simulink model "HvCoorn"  (R2022b)
settings: configuration reference "Icar05FusaMdlCfg" (kept outside this file)
undefined symbols (not defined in the file): BMSActSt_ACChrg, BMSActSt_DCChrg, BMSActSt_disconnect, BMSActSt_offline, BMSActSt_online, BMSActSt_undefined, BMSMainNegRlySt_Clsd_SC, BMSMainNegRlySt_Open_SC, BMSMainNegRlySt_StuckInClsd_SC, BMSMainNegRlySt_StuckInOpen_SC, BMSMainPosRlySt_Clsd_SC, BMSMainPosRlySt_Open_SC, BMSMainPosRlySt_StuckInClsd_SC, BMSPrecRlySt_StuckInOpen_SC, BMSReqSt_ACChrg, BMSReqSt_DCChrg, BMSReqSt_emergencyOffline, BMSReqSt_offline, BMSReqSt_online, Chrg_stCycleBookMod_SC, Chrg_stSingleBookMod_SC, CmpgMod_stInactv_SC, DCDCActSt_buck, DCDCActSt_connected, DCDCActSt_disconnected, DCDCReqSt_buck, DCDCReqSt_standby, EngStrtStop_RefuModDft_SC, EPBActSt_Appld_SC, GearLvr_stDrvGearD_SC, GearLvr_stDrvGearN_SC, GearLvr_stDrvGearP_SC, GearLvr_stDrvGearR_SC, hpp_bACChargeLinkIni_C, hpp_bACChargeLinkOKIni_C, hpp_bAcChgEnaIni_C, hpp_bAcChgPauseIni_C, hpp_bAcLinkTempErrIni_C, hpp_bBattWarmReqIni_C, hpp_bHvilHwErrIni_C, hpp_bHvilStOkIni_C, hpp_bHvRelayClsActIni_C, hpp_bHvRelayOpnActIni_C, hpp_bHvRelayStuckIni_C, hpp_bParked4ChDchgIni_C, hpp_bRemLvBatMntnReqIni_C, hpp_bStartUpReqIni_C, hpp_stHvilCanIni_C, hpp_stWarmTimeCfgRespIni_C, HvCoorn_bAuthEnaSwt_C, HvCoorn_bAuthFailSpdLimOvrd_C, HvCoorn_bAuthFailSpdLimOvrdVal_C, HvCoorn_bAuthStrt_C, HvCoorn_bBMSUnexpdDcnctFailEna_C, HvCoorn_bBuck2RdyBypDCDCEna_C, HvCoorn_bDCChrgFctCfg_C, HvCoorn_bDcChrgWkupEnaChrgLink_C, HvCoorn_bDCDcnct4ACEna_C, HvCoorn_bDCNotBuck2ShtdwnEna_C, HvCoorn_bDrvrLevNotRdyEna_C ... (+295)
libraries: ITKLib x213, simulink x61
(part 2 of 12)

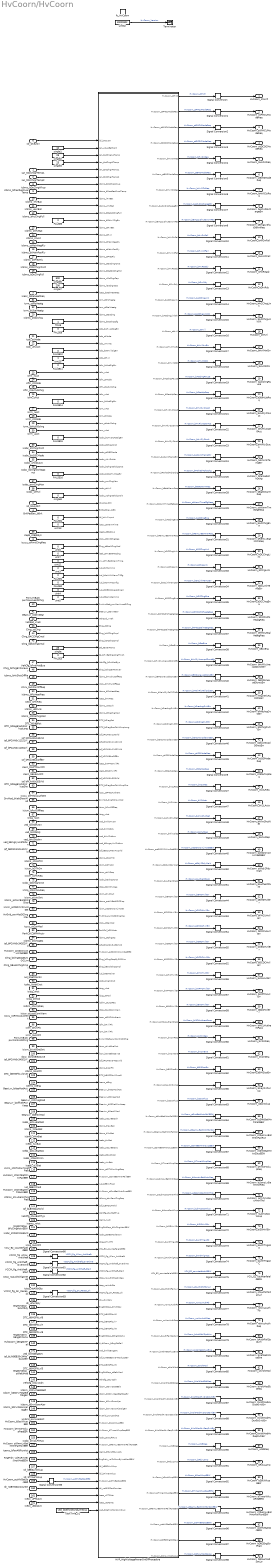
== system HvCoorn/HvCoorn ==
  ian_tDcChrgrTemp1 : Inport  OutDataTypeStr=single  Unit=deg
  ian_tDcChrgrTemp2 : Inport  Port=2  OutDataTypeStr=single  Unit=deg
  iczcu_stRmtChrgReq : Inport  Port=3  Unit=flg
  BrkPedDev_bBrk : Inport  Port=4  OutDataTypeStr=boolean  Unit=flg
  idi_bKeyStrt : Inport  Port=5  OutDataTypeStr=boolean  Unit=flg
  idi_bKeyOn : Inport  Port=6  OutDataTypeStr=boolean  Unit=flg
  icecc_bStalHeatReq : Inport  Port=7  OutDataTypeStr=boolean
  icbms_bDcChrgWkup : Inport  Port=8  OutDataTypeStr=boolean  Unit=flg
  icbms_bPrecResOverTemp : Inport  Port=9  OutDataTypeStr=boolean  Unit=flg
  icbms_iHVBat : Inport  Port=10  OutDataTypeStr=single  Unit=A
  icbms_uHVBat : Inport  Port=11  OutDataTypeStr=single  Unit=V
  icbms_bAcChrgFull : Inport  Port=12  OutDataTypeStr=boolean  Unit=flg
  icbms_stHvBat : Inport  Port=13  OutDataTypeStr=uint8
  icbms_stHvil : Inport  Port=14  OutDataTypeStr=uint8
  icbms_stMainNegRly : Inport  Port=15  OutDataTypeStr=uint8
  icbms_stMainPosRly : Inport  Port=16  OutDataTypeStr=uint8
  icbms_stPrecRly : Inport  Port=17  OutDataTypeStr=uint8
  icbms_stDcChrgrCnct : Inport  Port=18  OutDataTypeStr=uint8
  icbms_bDcChrgFull : Inport  Port=19  OutDataTypeStr=boolean  Unit=flg
  icbms_stDcChrg : Inport  Port=20
  icdc_stMode : Inport  Port=21  OutDataTypeStr=uint8
  icdc_uHvAct : Inport  Port=22  OutDataTypeStr=single  Unit=V
  icfm_nAct : Inport  Port=23  OutDataTypeStr=single  Unit=rpm
  icfm_stMode : Inport  Port=24  OutDataTypeStr=uint8
  icfm_stActvDchrg : Inport  Port=25  OutDataTypeStr=uint8
  icfm_uAct : Inport  Port=26  OutDataTypeStr=single  Unit=V
  icrm_nAct : Inport  Port=27  OutDataTypeStr=single  Unit=rpm
  icrm_stMode : Inport  Port=28  OutDataTypeStr=uint8
  icrm_stActvDchrg : Inport  Port=29  OutDataTypeStr=uint8
  icrm_uAct : Inport  Port=30  OutDataTypeStr=single  Unit=V
  icrm_stPlsHeatg : Inport  Port=31  OutDataTypeStr=uint8
  icrm_stStalHeatg : Inport  Port=32  OutDataTypeStr=uint8
  icobc_stChrgrCnct : Inport  Port=33  OutDataTypeStr=uint8
  icobc_stOBCMode : Inport  Port=34  OutDataTypeStr=uint8
  icobc_uHvDcAct : Inport  Port=35  OutDataTypeStr=single  Unit=V
  icobc_bChrgrCtrlSigCnct : Inport  Port=36
  icobc_pwrChrgMax : Inport  Port=37  OutDataTypeStr=single  Unit=W
  icobc_stHvil : Inport  Port=38  OutDataTypeStr=uint8
  icepb_stEpbSys : Inport  Port=39  OutDataTypeStr=uint8
  PwrLimBatt_pwrMaxHvesDChrg : Inport  Port=40  OutDataTypeStr=single  Unit=W
  GearLvr_stDrvGear : Inport  Port=41  OutDataTypeStr=uint8
  VehSpd_vVeh : Inport  Port=42  OutDataTypeStr=single  Unit=kph
  Chrg_stChrg : Inport  Port=43  OutDataTypeStr=uint8
  Chrg_bACChrgCmpl : Inport  Port=44  OutDataTypeStr=boolean  Unit=flg
  Chrg_bDCChrgCmpl : Inport  Port=45  OutDataTypeStr=boolean  Unit=flg
  Chrg_bChrgErrForever : Inport  Port=46  OutDataTypeStr=boolean  Unit=flg
  VehCfg_bFrntMotByp : Inport  Port=47  Unit=enum
  icbms_bHvShutOffReq : Inport  Port=48
  iczcu_bHVPwrOffReq : Inport  Port=49  OutDataTypeStr=boolean  Unit=flg
  icbms_bPlsHeatReq : Inport  Port=50
  icecc_bHVReq : Inport  Port=51
  icbms_uDCLnk : Inport  Port=52
  icbms_stPrechrgMod : Inport  Port=53
  DTC_bDiagRst : Inport  Port=54
  DTC_bDiagEnaCdnWkupLong : Inport  Port=55
  ipf_bPCAN0x130Vld : Inport  Port=56
  ipf_bPCAN0x111S1Vld : Inport  Port=57
  ipf_bPCAN0x110S1Vld : Inport  Port=58
  ipf_bPCANBusOffErr : Inport  Port=59
  icecc_bWPTCHvilFlt : Inport  Port=60
  icecc_bEASHvilFlt : Inport  Port=61
  ipf_bPCAN0x353Vld : Inport  Port=62
  DTC_bDiagEnaCdnWkupSho : Inport  Port=63
  iczcu_stFMCUAuthent : Inport  Port=64
  DrvMod_bVehShowMod : Inport  Port=65
  icicm_bPwrOffReq : Inport  Port=66
  icisg_nAct : Inport  Port=67
  ved_bInhbHvOn : Inport  Port=68
  ved_bInhbRdy : Inport  Port=69
  ved_bHvShtdwn : Inport  Port=70
  ved_bEmgcyHvShtdwn : Inport  Port=71
  ipf_bBD1CAN0x41CVld : Inport  Port=72
  icbms_stIsolTst : Inport  Port=73
  icicm_bOTAOn : Inport  Port=74
  icicm_stHVReq : Inport  Port=75
  icobc_bDchrgrCnct : Inport  Port=76
  ictcp_stRmtHvReq : Inport  Port=77
  icicm_stIvtrSwt : Inport  Port=78
  icbms_pctHVBatSOCDisp : Inport  Port=79
  icicm_pctSOCV2XLimSet : Inport  Port=80
  HvGrid_pwrMotDChrgMax : Inport  Port=81
  iczcu_stCarMod : Inport  Port=82
  ParkCtrl_bRPAActv : Inport  Port=83
  icbms_stChrgSts : Inport  Port=84
  ipf_bPCAN0x343S2Vld : Inport  Port=85
  HvCoorn_pctSOCV2XLimSetEER : Inport  Port=86
  Chrg_bChrgStopBySOCLim : Inport  Port=87
  Chrg_bBookChrgCmpl : Inport  Port=88
  iud_bNetMaintn : Inport  Port=89
  icobc_bVehCnct : Inport  Port=90
  icisg_uAct : Inport  Port=91
  icisg_stMod : Inport  Port=92
  icdkm_stLrcpReq : Inport  Port=93
  ictcp_stLostComWarn : Inport  Port=94
  iczcu_stRMCUAuthent : Inport  Port=95
  icfm_bHvilFlt : Inport  Port=96
  icrm_bHvilFlt : Inport  Port=97
  PwrLimBatt_pwrContnsDChrg : Inport  Port=98
  icicm_stIvtrEnaSwt : Inport  Port=99
  ibsw_bCnctElecDvce : Inport  Port=100
  ipf_bPCAN0x340S1Vld : Inport  Port=101
  icbms_bIsolFlt : Inport  Port=102
  DTC_bBMSFltLvlOver5 : Inport  Port=103
  icems_stEng : Inport  Port=104
  GearLvr_bNapModActv : Inport  Port=105
  GearLvr_stCmpgMod : Inport  Port=106
  GearLvr_bOffVehPwrKeep : Inport  Port=107
  GearLvr_bSentilMod : Inport  Port=108
  icebs_pctLvBatSoh : Inport  Port=109
  icbms_tMaxBat : Inport  Port=110
  icbms_tMinBat : Inport  Port=111
  icebs_tLvBat : Inport  Port=112
  icebs_pctLvBatSoc : Inport  Port=113
  icebs_stSocPrcsn : Inport  Port=114
  icebs_uLvBat : Inport  Port=115
  icicm_stOTAPwrMngtReq : Inport  Port=116
  HvCoorn_ctSmtBatMntnFailEER : Inport  Port=117
  iud_bEEIniFnsd : Inport  Port=118
  HvCoorn_ctSmtBatMntnSucsEER : Inport  Port=119
  iclbms_stLvRemChrgReq : Inport  Port=120
  ipf_bLBMSCANVld : Inport  Port=121
  VehCfg_stLvBattTyp : Inport  Port=122
  icems_nAct : Inport  Port=123
  EngStrtStop_bFuChrgActvEEW : Inport  Port=124
  icobc_stOBCModeV2In : Inport  Port=125
  icisg_bHvilFlt : Inport  Port=126
  VCU_E2_counterfaieldEER : Inport  Port=127
  VCCM_flg_Allow_Antitheft : Inport  Port=128
  VCCM_flg_Antitheft_Overtime : Inport  Port=129
  VCCM_flg_Antitheft_Start : Inport  Port=130
  ictcp_noAuthChlgOnReq : Inport  Port=131
  ictcp_noAuthSts : Inport  Port=132
  VCCM_flg_SK_Recep_ok : Inport  Port=133
  idi_uPwrSply : Inport  Port=134
  EngStrtStop_bHVPRdy : Inport  Port=135
  DTC_bBMSFltLvl6 : Inport  Port=136
  DTC_bBMSFltLvl7 : Inport  Port=137
  DTC_bBMSFltLvl8 : Inport  Port=138
  EngStrtStop_bEngStrtAllw : Inport  Port=139
  HybCoorn_bEngStrtFail : Inport  Port=140
  ved_bInhbEngStrt : Inport  Port=141
  ipf_bLIN9EBS0x34NodLostErr : Inport  Port=142
  DTC_bBMSFltLvl5 : Inport  Port=143
  EngStrtStop_stRefuMod : Inport  Port=144
  VehCfg_stCycCdn : Inport  Port=145
  icbcm_stDrvrSeatBelt : Inport  Port=146
  icbcm_bStDrvrSeatBeltSigErr : Inport  Port=147
  icbcm_bDrvrDoorAjar : Inport  Port=148
  icbcm_bDrvrDoorAjarSigErr : Inport  Port=149
  HvGrid_pwrLoadAct : Inport  Port=150
  HvCoorn_bSocWkupEER : Inport  Port=151
  HvCoorn_bTimerWkupReqEER : Inport  Port=152
  icobc_stV2LFltTyp : Inport  Port=153
  HvCoorn_stRemLvBatMntnFailRsnEER : Inport  Port=154
  icems_bFanAftRunActv : Inport  Port=155
  RngPrdn_volFuRmnByInstModEEW : Inport  Port=156
  idi_bEBSLinWkup : Inport  Port=157
  idi_bTimerWkup : Inport  Port=158
  HvCoorn_pctHVBatSocEER : Inport  Port=159
  idi_noBMSSocCounter : Inport  Port=160
  icecc_uPTCAct : Inport  Port=161
  icecc_uEASAct : Inport  Port=162
  fc_HvCoorn : TriggerPort  TriggerType=function-call  VariantControl=(inherit)
  FALSE{1..5,8,10..11,14..16} (11 alike) : Constant  Description=FALSE  Value=0  OutDataTypeStr=boolean
      settings: AttributesFormatString=%<Description>
  HVP_HighVoltagePowerOnOffProcedure : Subsystem
  Signal Conversion{,1..98} (99 alike) : SignalConversion  OverrideOpt=off
  TRUE : Constant  Description=TRUE  OutDataTypeStr=boolean
      settings: AttributesFormatString=%<Description>
  TaskTime_s1 : Constant  Description=[4]  Value=ved_bCellVoltUndLimSrus  SampleTime=-1
      settings: AttributesFormatString=%<Description>
  Terminator : Terminator
  single : Constant  Value=25  OutDataTypeStr=single
      settings: AttributesFormatString=%<OutDataTypeStr>
  single1 : Constant  Value=12  OutDataTypeStr=single
      settings: AttributesFormatString=%<OutDataTypeStr>
  single2 : Constant  Value=25  OutDataTypeStr=single
      settings: AttributesFormatString=%<OutDataTypeStr>
  single3 : Constant  Value=25  OutDataTypeStr=single
      settings: AttributesFormatString=%<OutDataTypeStr>
  single6 : Constant  Value=500  OutDataTypeStr=single
      settings: AttributesFormatString=%<OutDataTypeStr>
  single7 : Constant  Value=200  OutDataTypeStr=single
      settings: AttributesFormatString=%<OutDataTypeStr>
  single8 : Constant  Value=0  OutDataTypeStr=single
      settings: AttributesFormatString=%<OutDataTypeStr>
  uint{4,6..7,11,13} (5 alike) : Constant  Value=0  OutDataTypeStr=uint8
      settings: AttributesFormatString=%<OutDataTypeStr>
  uint25 : Constant  Description=DCDCClosed  OutDataTypeStr=uint8
      settings: AttributesFormatString=|
      | %<OutDataTypeStr>
      | %<Description>
  uint3 : Constant  Value=2  OutDataTypeStr=uint8
      settings: AttributesFormatString=%<OutDataTypeStr>
  uint32 : Constant  Value=10020302  OutDataTypeStr=uint32  SampleTime=-1
      settings: AttributesFormatString=%<OutDataTypeStr>
  uint5 : Constant  Value=2  OutDataTypeStr=uint8
      settings: AttributesFormatString=%<OutDataTypeStr>
  HvCoorn_stHVP : Outport
  HvCoorn_stFMCUModeReq : Outport  Port=2
  HvCoorn_stRMCUModeReq : Outport  Port=3
  HvCoorn_stDCDCModeReq : Outport  Port=4
  HvCoorn_bHvOnReq : Outport  Port=5
  HvCoorn_stBMSModeReq : Outport  Port=6
  HvCoorn_bHvilClsReq : Outport  Port=7
  HvCoorn_bActvDischargeErr : Outport  Port=8
  HvCoorn_bEmgcyShutDownReq : Outport  Port=9
  HvCoorn_bHvOnFail : Outport  Port=10
  HvCoorn_bHvInitFail : Outport  Port=11
  HvCoorn_bHvReady : Outport  Port=12
  HvCoorn_bDrvRdy : Outport  Port=13
  HvCoorn_bACChrgLink : Outport  Port=14
  HvCoorn_bACChrgLinkOk : Outport  Port=15
  HvCoorn_stHvil : Outport  Port=16
  HvCoorn_bHvilHwErr : Outport  Port=17
  HvCoorn_bHvilStOk : Outport  Port=18
  HvCoorn_bACChrgPause : Outport  Port=19
  HvCoorn_bStartUpReq : Outport  Port=20
  HvCoorn_bHvRlyClsAct : Outport  Port=21
  HvCoorn_bHvRlyOpenAct : Outport  Port=22
  HvCoorn_bHvRlyStuck : Outport  Port=23
  HvCoorn_bACLinkTempErr : Outport  Port=24
  HvCoorn_bParked4ChDchg : Outport  Port=25
  HvCoorn_bBattWarmReq : Outport  Port=26
  HvCoorn_stWarmTimeCfgResp : Outport  Port=27
  HvCoorn_bACChrgEna : Outport  Port=28
  HvCoorn_bRemLvBatMntnReq : Outport  Port=29
  HvCoorn_bDCChrgLink : Outport  Port=30
  HvCoorn_bChrgLink : Outport  Port=31
  HvCoorn_bDCLinkTempErr : Outport  Port=32
  HvCoorn_bDCChrgEna : Outport  Port=33
  HvCoorn_bRMCUPlsHeatgReq : Outport  Port=34
  HvCoorn_bRMCUStalHeatgReq : Outport  Port=35
  HvCoorn_bEccEna : Outport  Port=36
  HvCoorn_bHvRlyUnexpdDcnctErr : Outport  Port=37
  HvCoorn_bBMSUnexpdDcnctErr : Outport  Port=38
  HvCoorn_bMainRlyFail2ClsErr : Outport  Port=39
  HvCoorn_bPrechrgOvtiErr : Outport  Port=40
  HvCoorn_bDchrgOvtiErr : Outport  Port=41
  HvCoorn_bDCUnexpdDcnctErr : Outport  Port=42
  HvCoorn_stISGModeReq : Outport  Port=43
  HvCoorn_stStartUpReq : Outport  Port=44  VectorParamsAs1DForOutWhenUnconnected=off
  HvCoorn_bV2LReq : Outport  Port=45
  HvCoorn_bV2LActv : Outport  Port=46
  HvCoorn_bAllwShutNet : Outport  Port=47
  HvCoorn_bAllwSlep : Outport  Port=48
  HvCoorn_pctSOCV2XLimSetEEW : Outport  Port=49
  HvCoorn_stRdy2RdyWait : Outport  Port=50  VectorParamsAs1DForOutWhenUnconnected=off
  HvCoorn_bAuthentPass : Outport  Port=51  VectorParamsAs1DForOutWhenUnconnected=off
  HvCoorn_bBMSHvilErr : Outport  Port=52  VectorParamsAs1DForOutWhenUnconnected=off
  HvCoorn_bFMCUHvilErr : Outport  Port=53  VectorParamsAs1DForOutWhenUnconnected=off
  HvCoorn_bRMCUHvilErr : Outport  Port=54  VectorParamsAs1DForOutWhenUnconnected=off
  HvCoorn_bOBCHvilErr : Outport  Port=55  VectorParamsAs1DForOutWhenUnconnected=off
  HvCoorn_bDCDCHvilErr : Outport  Port=56  VectorParamsAs1DForOutWhenUnconnected=off
  HvCoorn_bHWHvilErr : Outport  Port=57  VectorParamsAs1DForOutWhenUnconnected=off
  HvCoorn_bWPTCHvilErr : Outport  Port=58  VectorParamsAs1DForOutWhenUnconnected=off
  HvCoorn_bEASHvilErr : Outport  Port=59  VectorParamsAs1DForOutWhenUnconnected=off
  HvCoorn_bMCUAuthentPass : Outport  Port=60  VectorParamsAs1DForOutWhenUnconnected=off
  HvCoorn_bV2InReq : Outport  Port=61  VectorParamsAs1DForOutWhenUnconnected=off
  HvCoorn_bV2InEna : Outport  Port=62  VectorParamsAs1DForOutWhenUnconnected=off
  HvCoorn_bBMSIsoErr : Outport  Port=63  VectorParamsAs1DForOutWhenUnconnected=off
  HvCoorn_bKeyOnPwrUp : Outport  Port=64  VectorParamsAs1DForOutWhenUnconnected=off
  HvCoorn_bSocWkup : Outport  Port=65  VectorParamsAs1DForOutWhenUnconnected=off
  HvCoorn_ctSmtBatMntnFailEEW : Outport  Port=66  VectorParamsAs1DForOutWhenUnconnected=off
  HvCoorn_stRemLvBatMntnFailRsn : Outport  Port=67  VectorParamsAs1DForOutWhenUnconnected=off
  HvCoorn_ctSmtBatMntnSucsEEW : Outport  Port=68  VectorParamsAs1DForOutWhenUnconnected=off
  HvCoorn_bTimerWkupReq : Outport  Port=69  VectorParamsAs1DForOutWhenUnconnected=off
  HvCoorn_bLbmsLvBatMntnReq : Outport  Port=70  VectorParamsAs1DForOutWhenUnconnected=off
  HvCoorn_pctLbmsSocMntnThd : Outport  Port=71  VectorParamsAs1DForOutWhenUnconnected=off
  HvCoorn_bLbmsSocWkup : Outport  Port=72  VectorParamsAs1DForOutWhenUnconnected=off
  HvCoorn_bISGHvilErr : Outport  Port=73  VectorParamsAs1DForOutWhenUnconnected=off
  HvCoorn_bAntiTrig430 : Outport  Port=74  VectorParamsAs1DForOutWhenUnconnected=off
  HvCoorn_bAntiTrig42C : Outport  Port=75  VectorParamsAs1DForOutWhenUnconnected=off
  VCU_E2_counterfaieldEEW : Outport  Port=76  VectorParamsAs1DForOutWhenUnconnected=off
  HvCoorn_stAuthChkFailLvl : Outport  Port=77  VectorParamsAs1DForOutWhenUnconnected=off
  HvCoorn_noVcuAuthFb : Outport  Port=78  VectorParamsAs1DForOutWhenUnconnected=off
  HvCoorn_noVcuAuthReq : Outport  Port=79  VectorParamsAs1DForOutWhenUnconnected=off
  HvCoorn_bAuthFailSpdLim : Outport  Port=80  VectorParamsAs1DForOutWhenUnconnected=off
  HvCoorn_bVehNetWkupEna : Outport  Port=81  VectorParamsAs1DForOutWhenUnconnected=off
  HvCoorn_stVoltMod : Outport  Port=82  VectorParamsAs1DForOutWhenUnconnected=off
  HvCoorn_bVoltModStbReq : Outport  Port=83  VectorParamsAs1DForOutWhenUnconnected=off
  HvCoorn_bVoltModHvDisbOvtiErr : Outport  Port=84  VectorParamsAs1DForOutWhenUnconnected=off
  HvCoorn_bVoltModHvDcnctOvtiErr : Outport  Port=85  VectorParamsAs1DForOutWhenUnconnected=off
  HvCoorn_bVoltModHvReqOvtiErr : Outport  Port=86  VectorParamsAs1DForOutWhenUnconnected=off
  HvCoorn_uISGReq : Outport  Port=87  VectorParamsAs1DForOutWhenUnconnected=off
  HvCoorn_bRdyLamp : Outport  Port=88
  HvCoorn_bSocWkupEEW : Outport  Port=89  VectorParamsAs1DForOutWhenUnconnected=off
  HvCoorn_bTimerWkupReqEEW : Outport  Port=90  VectorParamsAs1DForOutWhenUnconnected=off
  HvCoorn_stRemLvBatMntnFailRsnEEW : Outport  Port=91  VectorParamsAs1DForOutWhenUnconnected=off
  HvCoorn_pctHVBatSocEEW : Outport  Port=92  VectorParamsAs1DForOutWhenUnconnected=off
  HvCoorn_bDft2EngStrtRaw : Outport  Port=93  VectorParamsAs1DForOutWhenUnconnected=off
  HvCoorn_bShowModSocLo : Outport  Port=94  VectorParamsAs1DForOutWhenUnconnected=off
  wires:
  icdc_stMode/1 -> HVP_HighVoltagePowerOnOffProcedure/28(icdc_stMode)
  icepb_stEpbSys/1 -> HVP_HighVoltagePowerOnOffProcedure/55(icepb_stEpbSys)
  icbms_stHvBat/1 -> HVP_HighVoltagePowerOnOffProcedure/13(icbms_stHvBat)
  icfm_stMode/1 -> HVP_HighVoltagePowerOnOffProcedure/34(icfm_stMode)
  iczcu_stRmtChrgReq/1 -> HVP_HighVoltagePowerOnOffProcedure/56(iczcu_stRmtChrgReq)
  idi_bKeyStrt/1 -> HVP_HighVoltagePowerOnOffProcedure/51(idi_bKeyStrt)
  icfm_nAct/1 -> HVP_HighVoltagePowerOnOffProcedure/33(icfm_nAct)
  VehSpd_vVeh/1 -> HVP_HighVoltagePowerOnOffProcedure/67(VehSpd_vVeh)
  icobc_pwrChrgMax/1 -> HVP_HighVoltagePowerOnOffProcedure/48(icobc_pwrChrgMax)
  PwrLimBatt_pwrMaxHvesDChrg/1 -> HVP_HighVoltagePowerOnOffProcedure/65(PwrLimBatt_pwrMaxHvesDChrg)
  icbms_stMainPosRly/1 -> HVP_HighVoltagePowerOnOffProcedure/16(icbms_stMainPosRly)
  icobc_bChrgrCtrlSigCnct/1 -> HVP_HighVoltagePowerOnOffProcedure/46(icobc_bChrgrCtrlSigCnct)
  icobc_stHvil/1 -> HVP_HighVoltagePowerOnOffProcedure/49(icobc_stHvil)
  icbms_stHvil/1 -> HVP_HighVoltagePowerOnOffProcedure/14(icbms_stHvil)
  GearLvr_stDrvGear/1 -> HVP_HighVoltagePowerOnOffProcedure/66(GearLvr_stDrvGear)
  icbms_bPrecResOverTemp/1 -> HVP_HighVoltagePowerOnOffProcedure/8(icbms_bPrecResOverTemp)
  icobc_stChrgrCnct/1 -> HVP_HighVoltagePowerOnOffProcedure/43(icobc_stChrgrCnct)
  icbms_stPrecRly/1 -> HVP_HighVoltagePowerOnOffProcedure/17(icbms_stPrecRly)
  icfm_uAct/1 -> HVP_HighVoltagePowerOnOffProcedure/36(icfm_uAct)
  icobc_uHvDcAct/1 -> HVP_HighVoltagePowerOnOffProcedure/45(icobc_uHvDcAct)
  icbms_uHVBat/1 -> HVP_HighVoltagePowerOnOffProcedure/10(icbms_uHVBat)
  icobc_stOBCMode/1 -> HVP_HighVoltagePowerOnOffProcedure/44(icobc_stOBCMode)
  icdc_uHvAct/1 -> HVP_HighVoltagePowerOnOffProcedure/29(icdc_uHvAct)
  icbms_iHVBat/1 -> HVP_HighVoltagePowerOnOffProcedure/9(icbms_iHVBat)
  icecc_bStalHeatReq/1 -> HVP_HighVoltagePowerOnOffProcedure/22(icecc_bStalHeatReq)
  icbms_bDcChrgFull/1 -> HVP_HighVoltagePowerOnOffProcedure/19(icbms_bBatDCChrgFull)
  icrm_stActvDchrg/1 -> HVP_HighVoltagePowerOnOffProcedure/40(icrm_stActvDchrg)
  icrm_uAct/1 -> HVP_HighVoltagePowerOnOffProcedure/41(icrm_uAct)
  icbms_bDcChrgWkup/1 -> HVP_HighVoltagePowerOnOffProcedure/7(icbms_bDcChrgWkup)
  icbms_bAcChrgFull/1 -> HVP_HighVoltagePowerOnOffProcedure/11(icbms_bBatACChrgFull)
  icfm_stActvDchrg/1 -> HVP_HighVoltagePowerOnOffProcedure/35(icfm_stActvDchrg)
  VehCfg_bFrntMotByp/1 -> HVP_HighVoltagePowerOnOffProcedure/73(VehCfg_bFrntMotByp)
  icrm_stMode/1 -> HVP_HighVoltagePowerOnOffProcedure/39(icrm_stMode)
  Chrg_stChrg/1 -> HVP_HighVoltagePowerOnOffProcedure/68(Chrg_stChrg)
  icrm_nAct/1 -> HVP_HighVoltagePowerOnOffProcedure/38(icrm_nAct)
  icbms_stDcChrg/1 -> HVP_HighVoltagePowerOnOffProcedure/25(icbms_stDcChrg)
  ian_tDcChrgrTemp2/1 -> HVP_HighVoltagePowerOnOffProcedure/6(ian_tDcChrgrTemp2)
  icbms_stDcChrgrCnct/1 -> HVP_HighVoltagePowerOnOffProcedure/18(icbms_stDcChrgrCnct)
  icrm_stPlsHeatg/1 -> HVP_HighVoltagePowerOnOffProcedure/23(icrm_stPlsHeatg)
  icrm_stStalHeatg/1 -> HVP_HighVoltagePowerOnOffProcedure/24(icrm_stStalHeatg)
  ian_tDcChrgrTemp1/1 -> HVP_HighVoltagePowerOnOffProcedure/5(ian_tDcChrgrTemp1)
  BrkPedDev_bBrk/1 -> HVP_HighVoltagePowerOnOffProcedure/52(BrkPedDev_bBrk)
  idi_bKeyOn/1 -> HVP_HighVoltagePowerOnOffProcedure/1(idi_bKeyOn)
  Chrg_bDCChrgCmpl/1 -> HVP_HighVoltagePowerOnOffProcedure/70(Chrg_bDCChrgCmpl)
  Chrg_bChrgErrForever/1 -> HVP_HighVoltagePowerOnOffProcedure/74(Chrg_bChrgErrForever)
  icbms_stMainNegRly/1 -> HVP_HighVoltagePowerOnOffProcedure/15(icbms_stMainNegRly)
  Chrg_bACChrgCmpl/1 -> HVP_HighVoltagePowerOnOffProcedure/69(Chrg_bACChrgCmpl)
  icbms_bHvShutOffReq/1 -> HVP_HighVoltagePowerOnOffProcedure/75(icbms_bHvShutOffReq)
  iczcu_bHVPwrOffReq/1 -> HVP_HighVoltagePowerOnOffProcedure/76(iczcu_bHVPwrOffReq)
  icbms_bPlsHeatReq/1 -> HVP_HighVoltagePowerOnOffProcedure/77(icbms_bPlsHeatReq)
  icecc_bHVReq/1 -> HVP_HighVoltagePowerOnOffProcedure/78(icecc_bHVReq)
  uint32/1 -> Terminator/1  "HvCoorn_Version"
  icbms_uDCLnk/1 -> HVP_HighVoltagePowerOnOffProcedure/79(icbms_uDCLnk)
  icbms_stPrechrgMod/1 -> HVP_HighVoltagePowerOnOffProcedure/80(icbms_stPrechrgMod)
  DTC_bDiagRst/1 -> HVP_HighVoltagePowerOnOffProcedure/81(DTC_bDiagRst)
  DTC_bDiagEnaCdnWkupLong/1 -> HVP_HighVoltagePowerOnOffProcedure/82(DTC_bDiagEnaCdnWkupLong)
  ipf_bPCAN0x130Vld/1 -> HVP_HighVoltagePowerOnOffProcedure/83(ipf_bPCAN0x130Vld)
  ipf_bPCAN0x111S1Vld/1 -> HVP_HighVoltagePowerOnOffProcedure/84(ipf_bPCAN0x111S1Vld)
  ipf_bPCAN0x110S1Vld/1 -> HVP_HighVoltagePowerOnOffProcedure/85(ipf_bPCAN0x110S1Vld)
  HVP_HighVoltagePowerOnOffProcedure/1(HvCoorn_stHVP) -> Signal Conversion/1  "HvCoorn_stHVP"
  HVP_HighVoltagePowerOnOffProcedure/2(HvCoorn_stFMCUModeReq) -> Signal Conversion1/1  "HvCoorn_stFMCUModeReq"
  HVP_HighVoltagePowerOnOffProcedure/3(HvCoorn_stRMCUModeReq) -> Signal Conversion2/1  "HvCoorn_stRMCUModeReq"
  HVP_HighVoltagePowerOnOffProcedure/4(HvCoorn_stDCDCModeReq) -> Signal Conversion3/1  "HvCoorn_stDCDCModeReq"
  HVP_HighVoltagePowerOnOffProcedure/5(HvCoorn_bHvOnReq) -> Signal Conversion4/1  "HvCoorn_bHvOnReq"
  HVP_HighVoltagePowerOnOffProcedure/6(HvCoorn_stBMSModeReq) -> Signal Conversion5/1  "HvCoorn_stBMSModeReq"
  HVP_HighVoltagePowerOnOffProcedure/7(HvCoorn_bHvilClsReq) -> Signal Conversion6/1  "HvCoorn_bHvilClsReq"
  HVP_HighVoltagePowerOnOffProcedure/8(HvCoorn_bActvDischargeErr) -> Signal Conversion7/1  "HvCoorn_bActvDischargeErr"
  HVP_HighVoltagePowerOnOffProcedure/9(HvCoorn_bEmgcyShutDownReq) -> Signal Conversion8/1  "HvCoorn_bEmgcyShutDownReq"
  HVP_HighVoltagePowerOnOffProcedure/10(HvCoorn_bHvOnFail) -> Signal Conversion10/1  "HvCoorn_bHvOnFail"
  HVP_HighVoltagePowerOnOffProcedure/11(HvCoorn_bHvInitFail) -> Signal Conversion11/1  "HvCoorn_bHvInitFail"
  HVP_HighVoltagePowerOnOffProcedure/12(HvCoorn_bHvReady) -> Signal Conversion12/1  "HvCoorn_bHvReady"
  HVP_HighVoltagePowerOnOffProcedure/13(HvCoorn_bDrvRdy) -> Signal Conversion13/1  "HvCoorn_bDrvRdy"
  HVP_HighVoltagePowerOnOffProcedure/14(HvCoorn_bACChrgLink) -> Signal Conversion14/1  "HvCoorn_bACChrgLink"
  HVP_HighVoltagePowerOnOffProcedure/15(HvCoorn_bACChrgLinkOk) -> Signal Conversion15/1  "HvCoorn_bACChrgLinkOk"
  HVP_HighVoltagePowerOnOffProcedure/16(HvCoorn_stHvil) -> Signal Conversion16/1  "HvCoorn_stHvil"
  HVP_HighVoltagePowerOnOffProcedure/17(HvCoorn_bHvilHwErr) -> Signal Conversion17/1  "HvCoorn_bHvilHwErr"
  HVP_HighVoltagePowerOnOffProcedure/18(HvCoorn_bHvilStOk) -> Signal Conversion18/1  "HvCoorn_bHvilStOk"
  HVP_HighVoltagePowerOnOffProcedure/19(HvCoorn_bACChrgPause) -> Signal Conversion19/1  "HvCoorn_bACChrgPause"
  HVP_HighVoltagePowerOnOffProcedure/20(HvCoorn_bStartUpReq) -> Signal Conversion20/1  "HvCoorn_bStartUpReq"
  HVP_HighVoltagePowerOnOffProcedure/21(HvCoorn_bHvRlyClsAct) -> Signal Conversion21/1  "HvCoorn_bHvRlyClsAct"
  HVP_HighVoltagePowerOnOffProcedure/22(HvCoorn_bHvRlyOpenAct) -> Signal Conversion22/1  "HvCoorn_bHvRlyOpenAct"
  HVP_HighVoltagePowerOnOffProcedure/23(HvCoorn_bHvRlyStuck) -> Signal Conversion23/1  "HvCoorn_bHvRlyStuck"
  HVP_HighVoltagePowerOnOffProcedure/24(HvCoorn_bACLinkTempErr) -> Signal Conversion24/1  "HvCoorn_bACLinkTempErr"
  HVP_HighVoltagePowerOnOffProcedure/25(HvCoorn_bParked4ChDchg) -> Signal Conversion25/1  "HvCoorn_bParked4ChDchg"
  HVP_HighVoltagePowerOnOffProcedure/26(HvCoorn_bBattWarmReq) -> Signal Conversion28/1  "HvCoorn_bBattWarmReq"
  HVP_HighVoltagePowerOnOffProcedure/27(HvCoorn_stWarmTimeCfgResp) -> Signal Conversion29/1  "HvCoorn_stWarmTimeCfgResp"
  HVP_HighVoltagePowerOnOffProcedure/28(HvCoorn_bACChrgEna) -> Signal Conversion30/1  "HvCoorn_bACChrgEna"
  HVP_HighVoltagePowerOnOffProcedure/29(HvCoorn_bRemLvBatMntnReq) -> Signal Conversion31/1  "HvCoorn_bRemLvBatMntnReq"
  HVP_HighVoltagePowerOnOffProcedure/30(HvCoorn_bDCChrgLink) -> Signal Conversion32/1  "HvCoorn_bDCChrgLink"
  HVP_HighVoltagePowerOnOffProcedure/31(HvCoorn_bChrgLink) -> Signal Conversion33/1  "HvCoorn_bChrgLink"
  HVP_HighVoltagePowerOnOffProcedure/32(HvCoorn_bDCLinkTempErr) -> Signal Conversion34/1  "HvCoorn_bDCLinkTempErr"
  HVP_HighVoltagePowerOnOffProcedure/33(HvCoorn_bDCChrgEna) -> Signal Conversion35/1  "HvCoorn_bDCChrgEna"
  HVP_HighVoltagePowerOnOffProcedure/34(HvCoorn_bRMCUPlsHeatgReq) -> Signal Conversion36/1  "HvCoorn_bRMCUPlsHeatgReq"
  HVP_HighVoltagePowerOnOffProcedure/35(HvCoorn_bRMCUStalHeatgReq) -> Signal Conversion37/1  "HvCoorn_bRMCUStalHeatgReq"
  HVP_HighVoltagePowerOnOffProcedure/36(HvCoorn_bEccEna) -> Signal Conversion38/1  "HvCoorn_bEccEna"
  HVP_HighVoltagePowerOnOffProcedure/37(HvCoorn_bHvRlyUnexpdDcnctErr) -> Signal Conversion39/1  "HvCoorn_bHvRlyUnexpdDcnctErr"
  HVP_HighVoltagePowerOnOffProcedure/38(HvCoorn_bBMSUnexpdDcnctErr) -> Signal Conversion40/1  "HvCoorn_bBMSUnexpdDcnctErr"
  HVP_HighVoltagePowerOnOffProcedure/39(HvCoorn_bMainRlyFail2ClsErr) -> Signal Conversion41/1  "HvCoorn_bMainRlyFail2ClsErr"
  HVP_HighVoltagePowerOnOffProcedure/40(HvCoorn_bPrechrgOvtiErr) -> Signal Conversion42/1  "HvCoorn_bPrechrgOvtiErr"
  HVP_HighVoltagePowerOnOffProcedure/41(HvCoorn_bDchrgOvtiErr) -> Signal Conversion43/1  "HvCoorn_bDchrgOvtiErr"
  Signal Conversion43/1 -> HvCoorn_bDchrgOvtiErr/1
  Signal Conversion2/1 -> HvCoorn_stRMCUModeReq/1
  Signal Conversion4/1 -> HvCoorn_bHvOnReq/1
  Signal Conversion3/1 -> HvCoorn_stDCDCModeReq/1
  Signal Conversion5/1 -> HvCoorn_stBMSModeReq/1
  Signal Conversion7/1 -> HvCoorn_bActvDischargeErr/1
  Signal Conversion8/1 -> HvCoorn_bEmgcyShutDownReq/1
  Signal Conversion6/1 -> HvCoorn_bHvilClsReq/1
  Signal Conversion10/1 -> HvCoorn_bHvOnFail/1
  Signal Conversion11/1 -> HvCoorn_bHvInitFail/1
  Signal Conversion12/1 -> HvCoorn_bHvReady/1
  Signal Conversion13/1 -> HvCoorn_bDrvRdy/1
  Signal Conversion14/1 -> HvCoorn_bACChrgLink/1
  Signal Conversion15/1 -> HvCoorn_bACChrgLinkOk/1
  Signal Conversion16/1 -> HvCoorn_stHvil/1
  Signal Conversion1/1 -> HvCoorn_stFMCUModeReq/1
  Signal Conversion/1 -> HvCoorn_stHVP/1
  Signal Conversion19/1 -> HvCoorn_bACChrgPause/1
  Signal Conversion17/1 -> HvCoorn_bHvilHwErr/1
  Signal Conversion21/1 -> HvCoorn_bHvRlyClsAct/1
  Signal Conversion20/1 -> HvCoorn_bStartUpReq/1
  Signal Conversion18/1 -> HvCoorn_bHvilStOk/1
  Signal Conversion22/1 -> HvCoorn_bHvRlyOpenAct/1
  Signal Conversion23/1 -> HvCoorn_bHvRlyStuck/1
  Signal Conversion24/1 -> HvCoorn_bACLinkTempErr/1
  Signal Conversion25/1 -> HvCoorn_bParked4ChDchg/1
  Signal Conversion38/1 -> HvCoorn_bEccEna/1
  Signal Conversion37/1 -> HvCoorn_bRMCUStalHeatgReq/1
  Signal Conversion39/1 -> HvCoorn_bHvRlyUnexpdDcnctErr/1
  Signal Conversion40/1 -> HvCoorn_bBMSUnexpdDcnctErr/1
  Signal Conversion41/1 -> HvCoorn_bMainRlyFail2ClsErr/1
  Signal Conversion42/1 -> HvCoorn_bPrechrgOvtiErr/1
  Signal Conversion28/1 -> HvCoorn_bBattWarmReq/1
  Signal Conversion29/1 -> HvCoorn_stWarmTimeCfgResp/1
  Signal Conversion32/1 -> HvCoorn_bDCChrgLink/1
  Signal Conversion30/1 -> HvCoorn_bACChrgEna/1
  Signal Conversion31/1 -> HvCoorn_bRemLvBatMntnReq/1
  Signal Conversion33/1 -> HvCoorn_bChrgLink/1
  Signal Conversion34/1 -> HvCoorn_bDCLinkTempErr/1
  Signal Conversion35/1 -> HvCoorn_bDCChrgEna/1
  Signal Conversion36/1 -> HvCoorn_bRMCUPlsHeatgReq/1
  ipf_bPCANBusOffErr/1 -> HVP_HighVoltagePowerOnOffProcedure/86(ipf_bPCANBusOffErr)
  icecc_bWPTCHvilFlt/1 -> HVP_HighVoltagePowerOnOffProcedure/87(icecc_bWPTCHvilFlt)
  icecc_bEASHvilFlt/1 -> HVP_HighVoltagePowerOnOffProcedure/88(icecc_bEASHvilFlt)
  ipf_bPCAN0x353Vld/1 -> HVP_HighVoltagePowerOnOffProcedure/89(ipf_bPCAN0x353Vld)
  DTC_bDiagEnaCdnWkupSho/1 -> HVP_HighVoltagePowerOnOffProcedure/90(DTC_bDiagEnaCdnWkupSho)
  Signal Conversion46/1 -> HvCoorn_bDCUnexpdDcnctErr/1
  HVP_HighVoltagePowerOnOffProcedure/42(HvCoorn_bDCUnexpdDcnctErr) -> Signal Conversion46/1  "HvCoorn_bDCUnexpdDcnctErr"
  iczcu_stFMCUAuthent/1 -> HVP_HighVoltagePowerOnOffProcedure/91(iczcu_stFMCUAuthent)
  DrvMod_bVehShowMod/1 -> HVP_HighVoltagePowerOnOffProcedure/92(DrvMod_bVehShowMod)
  icicm_bPwrOffReq/1 -> HVP_HighVoltagePowerOnOffProcedure/93(icicm_bPwrOffReq)
  HVP_HighVoltagePowerOnOffProcedure/43(HvCoorn_stISGModeReq) -> Signal Conversion26/1  "HvCoorn_stISGModeReq"
  Signal Conversion26/1 -> HvCoorn_stISGModeReq/1
  icisg_nAct/1 -> HVP_HighVoltagePowerOnOffProcedure/94(icisg_nAct)
  ved_bInhbHvOn/1 -> HVP_HighVoltagePowerOnOffProcedure/95(ved_bInhbHvOn)
  ved_bInhbRdy/1 -> HVP_HighVoltagePowerOnOffProcedure/96(ved_bInhbRdy)
  ved_bHvShtdwn/1 -> HVP_HighVoltagePowerOnOffProcedure/97(ved_bHvShtdwn)
  ved_bEmgcyHvShtdwn/1 -> HVP_HighVoltagePowerOnOffProcedure/98(ved_bEmgcyHvShtdwn)
  ipf_bBD1CAN0x41CVld/1 -> HVP_HighVoltagePowerOnOffProcedure/99(ipf_bBD1CAN0x41CVld)
  icbms_stIsolTst/1 -> HVP_HighVoltagePowerOnOffProcedure/100(icbms_stIsolTst)
  icicm_bOTAOn/1 -> HVP_HighVoltagePowerOnOffProcedure/101(icicm_bOTAOn)
  icicm_stHVReq/1 -> HVP_HighVoltagePowerOnOffProcedure/102(icicm_stHVReq)
  icobc_bDchrgrCnct/1 -> HVP_HighVoltagePowerOnOffProcedure/103(icobc_bDchrgrCnct)
  HVP_HighVoltagePowerOnOffProcedure/44(HvCoorn_stStartUpReq) -> Signal Conversion9/1  "HvCoorn_stStartUpReq"
  Signal Conversion9/1 -> HvCoorn_stStartUpReq/1
  ictcp_stRmtHvReq/1 -> HVP_HighVoltagePowerOnOffProcedure/104(ictcp_stRmtHvReq)
  icicm_stIvtrSwt/1 -> HVP_HighVoltagePowerOnOffProcedure/105(icicm_stIvtrSwt)
  icbms_pctHVBatSOCDisp/1 -> HVP_HighVoltagePowerOnOffProcedure/106(icbms_pctHVBatSOCDisp)
  icicm_pctSOCV2XLimSet/1 -> HVP_HighVoltagePowerOnOffProcedure/107(icicm_pctSOCV2XLimSet)
  HvGrid_pwrMotDChrgMax/1 -> HVP_HighVoltagePowerOnOffProcedure/108(HvGrid_pwrMotDChrgMax)
  HVP_HighVoltagePowerOnOffProcedure/45(HvCoorn_bV2LReq) -> Signal Conversion27/1  "HvCoorn_bV2LReq"
  HVP_HighVoltagePowerOnOffProcedure/46(HvCoorn_bV2LActv) -> Signal Conversion47/1  "HvCoorn_bV2LActv"
  Signal Conversion27/1 -> HvCoorn_bV2LReq/1
  Signal Conversion47/1 -> HvCoorn_bV2LActv/1
  HVP_HighVoltagePowerOnOffProcedure/47(HvCoorn_bAllwShutNet) -> Signal Conversion48/1  "HvCoorn_bAllwShutNet"
  HVP_HighVoltagePowerOnOffProcedure/48(HvCoorn_bAllwSlep) -> Signal Conversion49/1  "HvCoorn_bAllwSlep"
  Signal Conversion48/1 -> HvCoorn_bAllwShutNet/1
  Signal Conversion49/1 -> HvCoorn_bAllwSlep/1
  iczcu_stCarMod/1 -> HVP_HighVoltagePowerOnOffProcedure/109(iczcu_stCarMod)
  ParkCtrl_bRPAActv/1 -> HVP_HighVoltagePowerOnOffProcedure/110(ParkCtrl_bRPAActv)
  icbms_stChrgSts/1 -> HVP_HighVoltagePowerOnOffProcedure/111(icbms_stChrgSts)
  ipf_bPCAN0x343S2Vld/1 -> HVP_HighVoltagePowerOnOffProcedure/112(ipf_bPCAN0x343S2Vld)
  HvCoorn_pctSOCV2XLimSetEER/1 -> HVP_HighVoltagePowerOnOffProcedure/113(HvCoorn_pctSOCV2XLimSetEER)
  HVP_HighVoltagePowerOnOffProcedure/49(HvCoorn_pctSOCV2XLimSetEEW) -> Signal Conversion45/1  "HvCoorn_pctSOCV2XLimSetEEW"
  Signal Conversion45/1 -> HvCoorn_pctSOCV2XLimSetEEW/1
  Chrg_bChrgStopBySOCLim/1 -> HVP_HighVoltagePowerOnOffProcedure/114(Chrg_bChrgStopBySOCLim)
  Chrg_bBookChrgCmpl/1 -> HVP_HighVoltagePowerOnOffProcedure/115(Chrg_bBookChrgCmpl)
  FALSE2/1 -> HVP_HighVoltagePowerOnOffProcedure/62(iud_bNoHVHConfig)
  FALSE1/1 -> HVP_HighVoltagePowerOnOffProcedure/61(iud_bNoHVHWarmTiCfg)
  uint3/1 -> HVP_HighVoltagePowerOnOffProcedure/60(iud_stVCUImmo)
  uint5/1 -> HVP_HighVoltagePowerOnOffProcedure/64(iud_stRemoteImmo)
  uint4/1 -> HVP_HighVoltagePowerOnOffProcedure/63(iud_stOBCWakeUpOrigin)
  single3/1 -> HVP_HighVoltagePowerOnOffProcedure/4(ian_tAcChrgrNTemp)
  single1/1 -> HVP_HighVoltagePowerOnOffProcedure/2(ian_uSupBattVolt)
  single2/1 -> HVP_HighVoltagePowerOnOffProcedure/3(ian_tAcChrgrL1Temp)
  uint7/1 -> HVP_HighVoltagePowerOnOffProcedure/58(ictel_stHvBatPrecdng)
  uint6/1 -> HVP_HighVoltagePowerOnOffProcedure/57(Chrg_stBookChrgMod)
  uint11/1 -> HVP_HighVoltagePowerOnOffProcedure/59(inv_stHvBattWarmTime)
  FALSE4/1 -> HVP_HighVoltagePowerOnOffProcedure/53(idi_bHvilInput)
  uint13/1 -> HVP_HighVoltagePowerOnOffProcedure/54(icacu_stWarmTime)
  FALSE5/1 -> HVP_HighVoltagePowerOnOffProcedure/12(icbms_bStHvilSigErr)
  single6/1 -> HVP_HighVoltagePowerOnOffProcedure/20(icbms_uDcChgrCap)
  single7/1 -> HVP_HighVoltagePowerOnOffProcedure/21(icbms_iDcChgrCap)
  TRUE/1 -> HVP_HighVoltagePowerOnOffProcedure/26(icbms_bDcChrgCfg)
  FALSE8/1 -> HVP_HighVoltagePowerOnOffProcedure/27(icdc_bUHvActSigErr)
  FALSE10/1 -> HVP_HighVoltagePowerOnOffProcedure/30(icdc_bStHvilSigErr)
  uint25/1 -> HVP_HighVoltagePowerOnOffProcedure/31(icdc_stHvil)
  FALSE11/1 -> HVP_HighVoltagePowerOnOffProcedure/32(icfm_bUActSigErr)
  FALSE14/1 -> HVP_HighVoltagePowerOnOffProcedure/37(icrm_bUActSigErr)
  FALSE15/1 -> HVP_HighVoltagePowerOnOffProcedure/42(icobc_bUHvDcActSigErr)
  FALSE16/1 -> HVP_HighVoltagePowerOnOffProcedure/47(icobc_bStAcHvilSigErr)
  single8/1 -> HVP_HighVoltagePowerOnOffProcedure/50(icobc_uChrgrCtrlSigVolt)
  single/1 -> HVP_HighVoltagePowerOnOffProcedure/71(std_tExterTemp)
  FALSE3/1 -> HVP_HighVoltagePowerOnOffProcedure/72(tcj_bHvBatPrecdngFinish)
  iud_bNetMaintn/1 -> HVP_HighVoltagePowerOnOffProcedure/116(iud_bNetMaintn)
  icobc_bVehCnct/1 -> HVP_HighVoltagePowerOnOffProcedure/117(icobc_bVehCnct)
  HVP_HighVoltagePowerOnOffProcedure/50(HvCoorn_stRdy2RdyWait) -> Signal Conversion50/1  "HvCoorn_stRdy2RdyWait"
  Signal Conversion50/1 -> HvCoorn_stRdy2RdyWait/1
  HVP_HighVoltagePowerOnOffProcedure/51(HvCoorn_bAuthentPass) -> Signal Conversion51/1  "HvCoorn_bAuthentPass"
  Signal Conversion51/1 -> HvCoorn_bAuthentPass/1
  icisg_uAct/1 -> HVP_HighVoltagePowerOnOffProcedure/118(icisg_uAct)
  icisg_stMod/1 -> HVP_HighVoltagePowerOnOffProcedure/119(icisg_stMod)
  icdkm_stLrcpReq/1 -> HVP_HighVoltagePowerOnOffProcedure/120(icdkm_stLrcpReq)
  ictcp_stLostComWarn/1 -> HVP_HighVoltagePowerOnOffProcedure/121(ictcp_stLostComWarn)
  HVP_HighVoltagePowerOnOffProcedure/52(HvCoorn_bBMSHvilErr) -> Signal Conversion44/1  "HvCoorn_bBMSHvilErr"
  HVP_HighVoltagePowerOnOffProcedure/53(HvCoorn_bFMCUHvilErr) -> Signal Conversion53/1  "HvCoorn_bFMCUHvilErr"
  HVP_HighVoltagePowerOnOffProcedure/54(HvCoorn_bRMCUHvilErr) -> Signal Conversion54/1  "HvCoorn_bRMCUHvilErr"
  HVP_HighVoltagePowerOnOffProcedure/55(HvCoorn_bOBCHvilErr) -> Signal Conversion55/1  "HvCoorn_bOBCHvilErr"
  HVP_HighVoltagePowerOnOffProcedure/56(HvCoorn_bDCDCHvilErr) -> Signal Conversion52/1  "HvCoorn_bDCDCHvilErr"
  HVP_HighVoltagePowerOnOffProcedure/57(HvCoorn_bHWHvilErr) -> Signal Conversion56/1  "HvCoorn_bHWHvilErr"
  Signal Conversion52/1 -> HvCoorn_bDCDCHvilErr/1
  Signal Conversion44/1 -> HvCoorn_bBMSHvilErr/1
  Signal Conversion54/1 -> HvCoorn_bRMCUHvilErr/1
  Signal Conversion53/1 -> HvCoorn_bFMCUHvilErr/1
  Signal Conversion56/1 -> HvCoorn_bHWHvilErr/1
  Signal Conversion55/1 -> HvCoorn_bOBCHvilErr/1
  HVP_HighVoltagePowerOnOffProcedure/58(HvCoorn_bWPTCHvilErr) -> Signal Conversion57/1  "HvCoorn_bWPTCHvilErr"
  HVP_HighVoltagePowerOnOffProcedure/59(HvCoorn_bEASHvilErr) -> Signal Conversion58/1  "HvCoorn_bEASHvilErr"
  Signal Conversion58/1 -> HvCoorn_bEASHvilErr/1
  Signal Conversion57/1 -> HvCoorn_bWPTCHvilErr/1
  iczcu_stRMCUAuthent/1 -> HVP_HighVoltagePowerOnOffProcedure/122(iczcu_stRMCUAuthent)
  icfm_bHvilFlt/1 -> HVP_HighVoltagePowerOnOffProcedure/123(icfm_bHvilFlt)
  icrm_bHvilFlt/1 -> HVP_HighVoltagePowerOnOffProcedure/124(icrm_bHvilFlt)
  HVP_HighVoltagePowerOnOffProcedure/60(HvCoorn_bMCUAuthentPass) -> Signal Conversion59/1  "HvCoorn_bMCUAuthentPass"
  Signal Conversion59/1 -> HvCoorn_bMCUAuthentPass/1
  PwrLimBatt_pwrContnsDChrg/1 -> HVP_HighVoltagePowerOnOffProcedure/125(PwrLimBatt_pwrContnsDChrg)
  icicm_stIvtrEnaSwt/1 -> HVP_HighVoltagePowerOnOffProcedure/126(icicm_stIvtrEnaSwt)
  ibsw_bCnctElecDvce/1 -> HVP_HighVoltagePowerOnOffProcedure/127(ibsw_bCnctElecDvce)
  HVP_HighVoltagePowerOnOffProcedure/61(HvCoorn_bV2InReq) -> Signal Conversion60/1  "HvCoorn_bV2InReq"
  HVP_HighVoltagePowerOnOffProcedure/62(HvCoorn_bV2InEna) -> Signal Conversion61/1  "HvCoorn_bV2InEna"
  Signal Conversion60/1 -> HvCoorn_bV2InReq/1
  Signal Conversion61/1 -> HvCoorn_bV2InEna/1
  ipf_bPCAN0x340S1Vld/1 -> HVP_HighVoltagePowerOnOffProcedure/128(ipf_bPCAN0x340S1Vld)
  icbms_bIsolFlt/1 -> HVP_HighVoltagePowerOnOffProcedure/129(icbms_bIsolFlt)
  DTC_bBMSFltLvlOver5/1 -> HVP_HighVoltagePowerOnOffProcedure/130(DTC_bBMSFltLvlOver5)
  HVP_HighVoltagePowerOnOffProcedure/63(HvCoorn_bBMSIsoErr) -> Signal Conversion62/1  "HvCoorn_bBMSIsoErr"
  Signal Conversion62/1 -> HvCoorn_bBMSIsoErr/1
  icems_stEng/1 -> HVP_HighVoltagePowerOnOffProcedure/131(icems_stEng)
  GearLvr_bNapModActv/1 -> HVP_HighVoltagePowerOnOffProcedure/132(GearLvr_bNapModActv)
  GearLvr_stCmpgMod/1 -> HVP_HighVoltagePowerOnOffProcedure/133(GearLvr_stCmpgMod)
  GearLvr_bOffVehPwrKeep/1 -> HVP_HighVoltagePowerOnOffProcedure/134(GearLvr_bOffVehPwrKeep)
  GearLvr_bSentilMod/1 -> HVP_HighVoltagePowerOnOffProcedure/135(GearLvr_bSentilMod)
  icebs_pctLvBatSoh/1 -> HVP_HighVoltagePowerOnOffProcedure/136(icebs_pctLvBatSoh)
  icbms_tMaxBat/1 -> HVP_HighVoltagePowerOnOffProcedure/137(icbms_tMaxBat)
  icbms_tMinBat/1 -> HVP_HighVoltagePowerOnOffProcedure/138(icbms_tMinBat)
  icebs_tLvBat/1 -> HVP_HighVoltagePowerOnOffProcedure/139(icebs_tLvBat)
  icebs_pctLvBatSoc/1 -> HVP_HighVoltagePowerOnOffProcedure/140(icebs_pctLvBatSoc)
  icebs_stSocPrcsn/1 -> HVP_HighVoltagePowerOnOffProcedure/141(icebs_stSocPrcsn)
  icebs_uLvBat/1 -> HVP_HighVoltagePowerOnOffProcedure/142(icebs_uLvBat)
  icicm_stOTAPwrMngtReq/1 -> HVP_HighVoltagePowerOnOffProcedure/143(icicm_stOTAPwrMngtReq)
  HvCoorn_ctSmtBatMntnFailEER/1 -> HVP_HighVoltagePowerOnOffProcedure/144(HvCoorn_ctSmtBatMntnFailEER)
  iud_bEEIniFnsd/1 -> HVP_HighVoltagePowerOnOffProcedure/145(iud_bEEIniFnsd)
  HVP_HighVoltagePowerOnOffProcedure/64(HvCoorn_bKeyOnPwrUp) -> Signal Conversion65/1
  HVP_HighVoltagePowerOnOffProcedure/65(HvCoorn_bSocWkup) -> Signal Conversion63/1  "HvCoorn_bSocWkup"
  HVP_HighVoltagePowerOnOffProcedure/66(HvCoorn_ctSmtBatMntnFailEEW) -> Signal Conversion64/1  "HvCoorn_ctSmtBatMntnFailEEW"
  Signal Conversion63/1 -> HvCoorn_bSocWkup/1
  Signal Conversion64/1 -> HvCoorn_ctSmtBatMntnFailEEW/1
  Signal Conversion65/1 -> HvCoorn_bKeyOnPwrUp/1
  HvCoorn_ctSmtBatMntnSucsEER/1 -> HVP_HighVoltagePowerOnOffProcedure/146(HvCoorn_ctSmtBatMntnSucsEER)
  HVP_HighVoltagePowerOnOffProcedure/67(HvCoorn_stRemLvBatMntnFailRsn) -> Signal Conversion66/1  "HvCoorn_stRemLvBatMntnFailRsn"
  HVP_HighVoltagePowerOnOffProcedure/68(HvCoorn_ctSmtBatMntnSucsEEW) -> Signal Conversion67/1  "HvCoorn_ctSmtBatMntnSucsEEW"
  Signal Conversion67/1 -> HvCoorn_ctSmtBatMntnSucsEEW/1
  Signal Conversion66/1 -> HvCoorn_stRemLvBatMntnFailRsn/1
  HVP_HighVoltagePowerOnOffProcedure/69(HvCoorn_bTimerWkupReq) -> Signal Conversion68/1  "HvCoorn_bTimerWkupReq"
  Signal Conversion68/1 -> HvCoorn_bTimerWkupReq/1
  iclbms_stLvRemChrgReq/1 -> HVP_HighVoltagePowerOnOffProcedure/147(iclbms_stLvRemChrgReq)
  ipf_bLBMSCANVld/1 -> HVP_HighVoltagePowerOnOffProcedure/148(ipf_bLBMSCANVld)
  VehCfg_stLvBattTyp/1 -> HVP_HighVoltagePowerOnOffProcedure/149(VehCfg_stLvBattTyp)
  HVP_HighVoltagePowerOnOffProcedure/70(HvCoorn_bLbmsLvBatMntnReq) -> Signal Conversion69/1  "HvCoorn_bLbmsLvBatMntnReq"
  HVP_HighVoltagePowerOnOffProcedure/71(HvCoorn_pctLbmsSocMntnThd) -> Signal Conversion70/1  "HvCoorn_pctLbmsSocMntnThd"
  HVP_HighVoltagePowerOnOffProcedure/72(HvCoorn_bLbmsSocWkup) -> Signal Conversion71/1  "HvCoorn_bLbmsSocWkup"
  Signal Conversion69/1 -> HvCoorn_bLbmsLvBatMntnReq/1
  Signal Conversion70/1 -> HvCoorn_pctLbmsSocMntnThd/1
  Signal Conversion71/1 -> HvCoorn_bLbmsSocWkup/1
  icems_nAct/1 -> HVP_HighVoltagePowerOnOffProcedure/150(icems_nAct)
  EngStrtStop_bFuChrgActvEEW/1 -> HVP_HighVoltagePowerOnOffProcedure/151(EngStrtStop_bFuChrgActvEEW)
  icobc_stOBCModeV2In/1 -> HVP_HighVoltagePowerOnOffProcedure/152(icobc_stOBCModeV2In)
  HVP_HighVoltagePowerOnOffProcedure/73(HvCoorn_bISGHvilErr) -> Signal Conversion72/1  "HvCoorn_bISGHvilErr"
  Signal Conversion72/1 -> HvCoorn_bISGHvilErr/1
  icisg_bHvilFlt/1 -> HVP_HighVoltagePowerOnOffProcedure/153(icisg_bHvilFlt)
  VCU_E2_counterfaieldEER/1 -> HVP_HighVoltagePowerOnOffProcedure/154(VCU_E2_counterfaieldEER)
  VCCM_flg_Allow_Antitheft/1 -> Signal Conversion80/1
  VCCM_flg_Antitheft_Overtime/1 -> Signal Conversion81/1
  VCCM_flg_Antitheft_Start/1 -> Signal Conversion82/1
  ictcp_noAuthChlgOnReq/1 -> HVP_HighVoltagePowerOnOffProcedure/158(ictcp_noAuthChlgOnReq)
  ictcp_noAuthSts/1 -> HVP_HighVoltagePowerOnOffProcedure/159(ictcp_noAuthSts)
  VCCM_flg_SK_Recep_ok/1 -> Signal Conversion83/1
  HVP_HighVoltagePowerOnOffProcedure/74(HvCoorn_bAntiTrig430) -> Signal Conversion73/1  "HvCoorn_bAntiTrig430"
  HVP_HighVoltagePowerOnOffProcedure/75(HvCoorn_bAntiTrig42C) -> Signal Conversion74/1  "HvCoorn_bAntiTrig42C"
  HVP_HighVoltagePowerOnOffProcedure/76(VCU_E2_counterfaieldEEW) -> Signal Conversion75/1  "VCU_E2_counterfaieldEEW"
  HVP_HighVoltagePowerOnOffProcedure/77(HvCoorn_stAuthChkFailLvl) -> Signal Conversion76/1  "HvCoorn_stAuthChkFailLvl"
  HVP_HighVoltagePowerOnOffProcedure/79(HvCoorn_noVcuAuthReq) -> Signal Conversion78/1  "HvCoorn_noVcuAuthReq"
  HVP_HighVoltagePowerOnOffProcedure/80(HvCoorn_bAuthFailSpdLim) -> Signal Conversion79/1  "HvCoorn_bAuthFailSpdLim"
  HVP_HighVoltagePowerOnOffProcedure/78(HvCoorn_noVcuAuthFb) -> Signal Conversion77/1  "HvCoorn_noVcuAuthFb"
  Signal Conversion74/1 -> HvCoorn_bAntiTrig42C/1
  Signal Conversion73/1 -> HvCoorn_bAntiTrig430/1
  Signal Conversion75/1 -> VCU_E2_counterfaieldEEW/1
  Signal Conversion77/1 -> HvCoorn_noVcuAuthFb/1
  Signal Conversion78/1 -> HvCoorn_noVcuAuthReq/1
  Signal Conversion76/1 -> HvCoorn_stAuthChkFailLvl/1
  Signal Conversion79/1 -> HvCoorn_bAuthFailSpdLim/1
  Signal Conversion80/1 -> HVP_HighVoltagePowerOnOffProcedure/155(VCCM_flg_Allow_Antitheft)  "VCCM_flg_Allow_Antitheft"
  Signal Conversion81/1 -> HVP_HighVoltagePowerOnOffProcedure/156(VCCM_flg_Antitheft_Overtime)  "VCCM_flg_Antitheft_Overtime"
  Signal Conversion82/1 -> HVP_HighVoltagePowerOnOffProcedure/157(VCCM_flg_Antitheft_Start)  "VCCM_flg_Antitheft_Start"
  Signal Conversion83/1 -> HVP_HighVoltagePowerOnOffProcedure/160(VCCM_flg_SK_Recep_ok)  "VCCM_flg_SK_Recep_ok"
  idi_uPwrSply/1 -> HVP_HighVoltagePowerOnOffProcedure/161(idi_uPwrSply)
  HVP_HighVoltagePowerOnOffProcedure/81(HvCoorn_bVehNetWkupEna) -> Signal Conversion84/1  "HvCoorn_bVehNetWkupEna"
  Signal Conversion84/1 -> HvCoorn_bVehNetWkupEna/1
  EngStrtStop_bHVPRdy/1 -> HVP_HighVoltagePowerOnOffProcedure/162(EngStrtStop_bHVPRdy)
  DTC_bBMSFltLvl6/1 -> HVP_HighVoltagePowerOnOffProcedure/163(DTC_bBMSFltLvl6)
  DTC_bBMSFltLvl7/1 -> HVP_HighVoltagePowerOnOffProcedure/164(DTC_bBMSFltLvl7)
  DTC_bBMSFltLvl8/1 -> HVP_HighVoltagePowerOnOffProcedure/165(DTC_bBMSFltLvl8)
  EngStrtStop_bEngStrtAllw/1 -> HVP_HighVoltagePowerOnOffProcedure/166(EngStrtStop_bEngStrtAllw)
  HybCoorn_bEngStrtFail/1 -> HVP_HighVoltagePowerOnOffProcedure/167(HybCoorn_bEngStrtFail)
  ved_bInhbEngStrt/1 -> HVP_HighVoltagePowerOnOffProcedure/168(ved_bInhbEngStrt)
  HVP_HighVoltagePowerOnOffProcedure/82(HvCoorn_stVoltMod) -> Signal Conversion85/1  "HvCoorn_stVoltMod"
  HVP_HighVoltagePowerOnOffProcedure/83(HvCoorn_bVoltModStbReq) -> Signal Conversion86/1  "HvCoorn_bVoltModStbReq"
  HVP_HighVoltagePowerOnOffProcedure/84(HvCoorn_bVoltModHvDisbOvtiErr) -> Signal Conversion87/1  "HvCoorn_bVoltModHvDisbOvtiErr"
  HVP_HighVoltagePowerOnOffProcedure/85(HvCoorn_bVoltModHvDcnctOvtiErr) -> Signal Conversion88/1  "HvCoorn_bVoltModHvDcnctOvtiErr"
  HVP_HighVoltagePowerOnOffProcedure/86(HvCoorn_bVoltModHvReqOvtiErr) -> Signal Conversion89/1  "HvCoorn_bVoltModHvReqOvtiErr"
  HVP_HighVoltagePowerOnOffProcedure/87(HvCoorn_uISGReq) -> Signal Conversion90/1  "HvCoorn_uISGReq"
  Signal Conversion87/1 -> HvCoorn_bVoltModHvDisbOvtiErr/1
  Signal Conversion88/1 -> HvCoorn_bVoltModHvDcnctOvtiErr/1
  Signal Conversion86/1 -> HvCoorn_bVoltModStbReq/1
  Signal Conversion89/1 -> HvCoorn_bVoltModHvReqOvtiErr/1
  Signal Conversion90/1 -> HvCoorn_uISGReq/1
  ipf_bLIN9EBS0x34NodLostErr/1 -> HVP_HighVoltagePowerOnOffProcedure/169(ipf_bLIN9EBS0x34NodLostErr)
  DTC_bBMSFltLvl5/1 -> HVP_HighVoltagePowerOnOffProcedure/170(DTC_bBMSFltLvl5)
  EngStrtStop_stRefuMod/1 -> HVP_HighVoltagePowerOnOffProcedure/171(EngStrtStop_stRefuMod)
  VehCfg_stCycCdn/1 -> HVP_HighVoltagePowerOnOffProcedure/172(VehCfg_stCycCdn)
  icbcm_stDrvrSeatBelt/1 -> HVP_HighVoltagePowerOnOffProcedure/173(icbcm_stDrvrSeatBelt)
  icbcm_bStDrvrSeatBeltSigErr/1 -> HVP_HighVoltagePowerOnOffProcedure/174(icbcm_bStDrvrSeatBeltSigErr)
  icbcm_bDrvrDoorAjar/1 -> HVP_HighVoltagePowerOnOffProcedure/175(icbcm_bDrvrDoorAjar)
  icbcm_bDrvrDoorAjarSigErr/1 -> HVP_HighVoltagePowerOnOffProcedure/176(icbcm_bDrvrDoorAjarSigErr)
  HVP_HighVoltagePowerOnOffProcedure/88(HvCoorn_bRdyLamp) -> Signal Conversion91/1  "HvCoorn_bRdyLamp"
  Signal Conversion91/1 -> HvCoorn_bRdyLamp/1
  HvGrid_pwrLoadAct/1 -> HVP_HighVoltagePowerOnOffProcedure/177(HvGrid_pwrLoadAct)
  HvCoorn_bSocWkupEER/1 -> HVP_HighVoltagePowerOnOffProcedure/178(HvCoorn_bSocWkupEER)
  HvCoorn_bTimerWkupReqEER/1 -> HVP_HighVoltagePowerOnOffProcedure/179(HvCoorn_bTimerWkupReqEER)
  HVP_HighVoltagePowerOnOffProcedure/89(HvCoorn_bSocWkupEEW) -> Signal Conversion92/1  "HvCoorn_bSocWkupEEW"
  HVP_HighVoltagePowerOnOffProcedure/90(HvCoorn_bTimerWkupReqEEW) -> Signal Conversion93/1  "HvCoorn_bTimerWkupReqEEW"
  Signal Conversion93/1 -> HvCoorn_bTimerWkupReqEEW/1
  Signal Conversion92/1 -> HvCoorn_bSocWkupEEW/1
  icobc_stV2LFltTyp/1 -> HVP_HighVoltagePowerOnOffProcedure/180(icobc_stV2LFltTyp)
  HvCoorn_stRemLvBatMntnFailRsnEER/1 -> HVP_HighVoltagePowerOnOffProcedure/181(HvCoorn_stRemLvBatMntnFailRsnEER)
  HVP_HighVoltagePowerOnOffProcedure/91(HvCoorn_stRemLvBatMntnFailRsnEEW) -> Signal Conversion94/1  "HvCoorn_stRemLvBatMntnFailRsnEEW"
  Signal Conversion94/1 -> HvCoorn_stRemLvBatMntnFailRsnEEW/1
  Signal Conversion85/1 -> HvCoorn_stVoltMod/1
  icems_bFanAftRunActv/1 -> HVP_HighVoltagePowerOnOffProcedure/182(icems_bFanAftRunActv)
  RngPrdn_volFuRmnByInstModEEW/1 -> HVP_HighVoltagePowerOnOffProcedure/183(RngPrdn_volFuRmnByInstModEEW)
  idi_bEBSLinWkup/1 -> HVP_HighVoltagePowerOnOffProcedure/184(idi_bEBSLinWkup)
  idi_bTimerWkup/1 -> HVP_HighVoltagePowerOnOffProcedure/185(idi_bTimerWkup)
  HvCoorn_pctHVBatSocEER/1 -> Signal Conversion95/1
  idi_noBMSSocCounter/1 -> HVP_HighVoltagePowerOnOffProcedure/187(idi_noBMSSocCounter)
  HVP_HighVoltagePowerOnOffProcedure/92(HvCoorn_pctHVBatSocEEW) -> Signal Conversion96/1  "HvCoorn_pctHVBatSocEEW"
  Signal Conversion95/1 -> HVP_HighVoltagePowerOnOffProcedure/186(HvCoorn_pctHVBatSocEER)  "HvCoorn_pctHVBatSocEER"
  Signal Conversion96/1 -> HvCoorn_pctHVBatSocEEW/1
  Signal Conversion97/1 -> HvCoorn_bDft2EngStrtRaw/1
  HVP_HighVoltagePowerOnOffProcedure/93(HvCoorn_bDft2EngStrtRaw) -> Signal Conversion97/1
  HVP_HighVoltagePowerOnOffProcedure/94(HvCoorn_bShowModSocLo) -> Signal Conversion98/1  "HvCoorn_bShowModSocLo"
  Signal Conversion98/1 -> HvCoorn_bShowModSocLo/1
  icecc_uPTCAct/1 -> HVP_HighVoltagePowerOnOffProcedure/188(icecc_uPTCAct)
  icecc_uEASAct/1 -> HVP_HighVoltagePowerOnOffProcedure/189(icecc_uEASAct)
  TaskTime_s1/1 -> HVP_HighVoltagePowerOnOffProcedure/190(ved_bCellVoltUndLimSrus)
